simulink model "BBW2_backup"  (Simulink 7.5)
settings: Solver=ode45  StartTime=0.0  StopTime=10.0  RelTol=1e-3
libraries: FunctionTypes x13
settings Model: Creator=ytp0142  LastModifiedBy=ytp0142

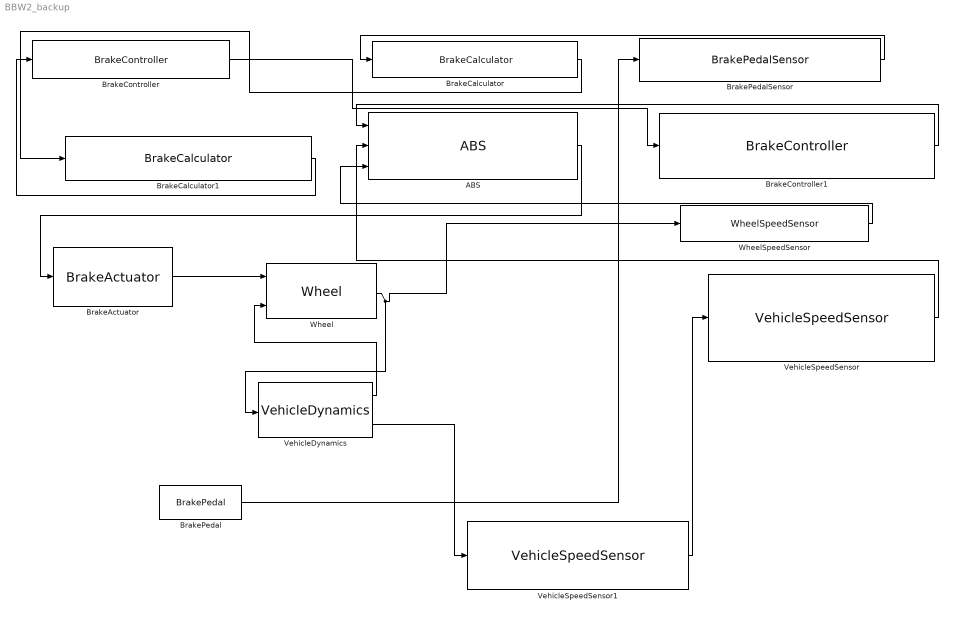
== system BBW2_backup ==
  ABS : FunctionTypes/ABS  SystemSampleTime=-1
  BrakeActuator : FunctionTypes/BrakeActuator  SystemSampleTime=-1
  BrakeCalculator : FunctionTypes/BrakeCalculator  SystemSampleTime=-1
  BrakeCalculator1 : FunctionTypes/BrakeCalculator  SystemSampleTime=-1
  BrakeController : FunctionTypes/BrakeController  SystemSampleTime=-1
  BrakeController1 : FunctionTypes/BrakeController  SystemSampleTime=-1
  BrakePedal : FunctionTypes/BrakePedal  SystemSampleTime=-1
  BrakePedalSensor : FunctionTypes/BrakePedalSensor  SystemSampleTime=-1
  VehicleDynamics : FunctionTypes/VehicleDynamics  SystemSampleTime=-1
  VehicleSpeedSensor : FunctionTypes/VehicleSpeedSensor  SystemSampleTime=-1
  VehicleSpeedSensor1 : FunctionTypes/VehicleSpeedSensor  SystemSampleTime=-1
  Wheel : FunctionTypes/Wheel  SystemSampleTime=-1
  WheelSpeedSensor : FunctionTypes/WheelSpeedSensor  SystemSampleTime=-1
  wires:
  BrakePedalSensor/1 -> BrakeCalculator/1
  WheelSpeedSensor/1 -> ABS/3
  ABS/1 -> BrakeActuator/1
  BrakeActuator/1 -> Wheel/1
  Wheel/1 -> VehicleDynamics/1, WheelSpeedSensor/1
  VehicleDynamics/1 -> Wheel/2
  VehicleSpeedSensor/1 -> ABS/2
  VehicleSpeedSensor1/1 -> VehicleSpeedSensor/1
  VehicleDynamics/2 -> VehicleSpeedSensor1/1
  BrakePedal/1 -> BrakePedalSensor/1
  BrakeCalculator/1 -> BrakeCalculator1/1
  BrakeCalculator1/1 -> BrakeController/1
  BrakeController/1 -> BrakeController1/1
  BrakeController1/1 -> ABS/1
